simulink subsystem "Polynomial_Filter"  (R2019b)
settings: Solver=VariableStepAuto  StartTime=0.0  StopTime=10.0  RelTol=1e-3
undefined symbols (not defined in the file): PARAMS
settings Model: Creator=opc  LastModifiedBy=opc

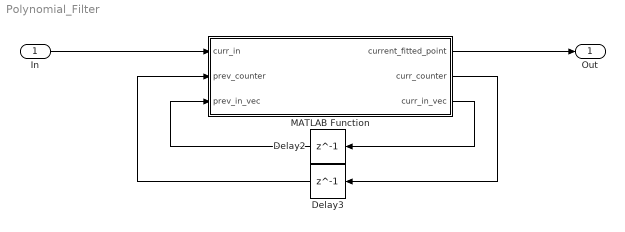
== system Polynomial_Filter ==
  In : Inport  PortDimensions=1
  Delay2 : Delay  DelayLength=1  InitialCondition=zeros(PARAMS.polyfit.window, 1)
  Delay3 : Delay  DelayLength=1  InitialCondition=0
  MATLAB Function : MATLAB Function  TreatAsAtomicUnit=on
  Out : Outport  PortDimensions=1
  wires:
  Delay3/1 -> MATLAB Function/2(prev_counter)
  MATLAB Function/3(curr_in_vec) -> Delay2/1
  In/1 -> MATLAB Function/1(curr_in)
  Delay2/1 -> MATLAB Function/3(prev_in_vec)
  MATLAB Function/2(curr_counter) -> Delay3/1
  MATLAB Function/1(current_fitted_point) -> Out/1

== matlab function Polynomial_Filter/MATLAB Function ==
  data: curr_in input size=1; prev_counter input size=1; current_fitted_point output size=1; curr_counter output size=1; prev_in_vec input size=PARAMS.polyfit.window; curr_in_vec output size=PARAMS.polyfit.window; PARAMS parameter
function [current_fitted_point, curr_counter, curr_in_vec] = fcn(curr_in, prev_counter, prev_in_vec, PARAMS)

curr_in_vec = [prev_in_vec(2:end); curr_in];
coeffs = PARAMS.polyfit.pinvR*((curr_in_vec - curr_in_vec(PARAMS.polyfit.center_idx)).*(PARAMS.polyfit.forgetting_factor.^((PARAMS.polyfit.window-1):-1:0)'));
data_reconstr = (repmat(PARAMS.polyfit.time, 1, length(coeffs)).^repmat(PARAMS.polyfit.powers, length(curr_in_vec), 1))*coeffs;
data_reconstr = data_reconstr + curr_in_vec(PARAMS.polyfit.center_idx);
curr_counter = prev_counter + 1;

if curr_counter > length(curr_in_vec)
    current_fitted_point = data_reconstr(end);
else
    current_fitted_point = curr_in;
end

end
